simulink model "TEST_SensorSource_Lookup"  (R2020b)
settings: Solver=ode1  StartTime=tspan(1)  StopTime=tspan(2)  FixedStep=1/sensorFs.imuUpdateFs  RelTol=1e-3
values from neighbouring files (symbols this model uses):
  mag1 = double([Sensors.mag1.mag_x, Sensors.mag1.mag_y, Sensors.mag1.mag_z])    [navi_marg22.m]    (also in navi_marg24.m; navi_mvo17.m)
  mag2 = double([Sensors.mag2.mag_x, Sensors.mag2.mag_y, Sensors.mag2.mag_z])    [navi_marg22.m]    (also in navi_marg24.m; navi_mvo17.m)
  time = naviRes.time    [Plot_NaviMARG.m]    (also in UAVPlotLib.m = sensors.(sensorName).time; myplot_navfilter.m = sensors.Algo.time_algo; myplot_sensor_filter_compare.m = sensors.IMU.time_imu; postplot_marg_flightdata.m = sensors.Algo.time_algo)
undefined symbols (not defined in the file or in its folder): airspeed1, airspeed2, airspeed3, baro1, IMU1, IMU1_Control, IMU2, IMU3, laserDown1, laserDown2, radar1, radarLongDown1, radarLongForward1, sensorFs, ublox1, um482
(part 1 of 2)
settings Model: PauseTimes=266.88  Creator=sl  LastModifiedBy=sl
settings SolverCC: AutoInsertRateTranBlk=on
settings OptimizationCC: DefaultParameterBehavior=Inlined  EnhancedBackFolding=on  PassReuseOutputArgsAs=Individual arguments  ZeroExternalMemoryAtStartup=off  ZeroInternalMemoryAtStartup=off  MaxStackSize=64  OptimizeBlockOrder=speed  DifferentSizesBufferReuse=on  OptimizationCustomize=off  EfficientTunableParamExpr=on
settings DebuggingCC: MultiTaskCondExecSysMsg=none  ParameterPrecisionLossMsg=none  ParameterTunabilityLossMsg=error  UnconnectedInputMsg=none  UnconnectedOutputMsg=none  UnconnectedLineMsg=none  BusObjectLabelMismatch=error
settings HardwareCC: ProdBitPerPointer=32  ProdBitPerSizeT=32  ProdBitPerPtrDiffT=32  ProdLargestAtomicInteger=Long  ProdLargestAtomicFloat=Double  ProdWordSize=32  ProdHWDeviceType=ARM Compatible->ARM Cortex
settings ModelReferenceCC: EnableParallelModelReferenceBuilds=on  ParallelModelReferenceMATLABWorkerInit=Load Top Model
settings SFSimCC: MATLABDynamicMemAlloc=off
settings RTWCC: Description=Embedded Coder  SystemTargetFile=ert.tlc  TemplateMakefile=ert_default_tmf  GenerateReport=on  Toolchain=GNU Tools for ARM Embedded Processors  IncludeHyperlinkInReport=on  LaunchReport=on  GenerateTraceInfo=on  GenerateTraceReport=on  GenerateTraceReportSl=on  GenerateTraceReportSf=on  GenerateTraceReportEml=on
settings CodeAppCC: ForceParamTrailComments=on  IgnoreCustomStorageClasses=off  OperatorAnnotations=on  SimulinkDataObjDesc=on  SFDataObjDesc=on  InsertBlockDesc=on
settings ERTTargetCC: InlinedParameterPlacement=NonHierarchical  ERTCustomFileTemplate=example_file_process.tlc

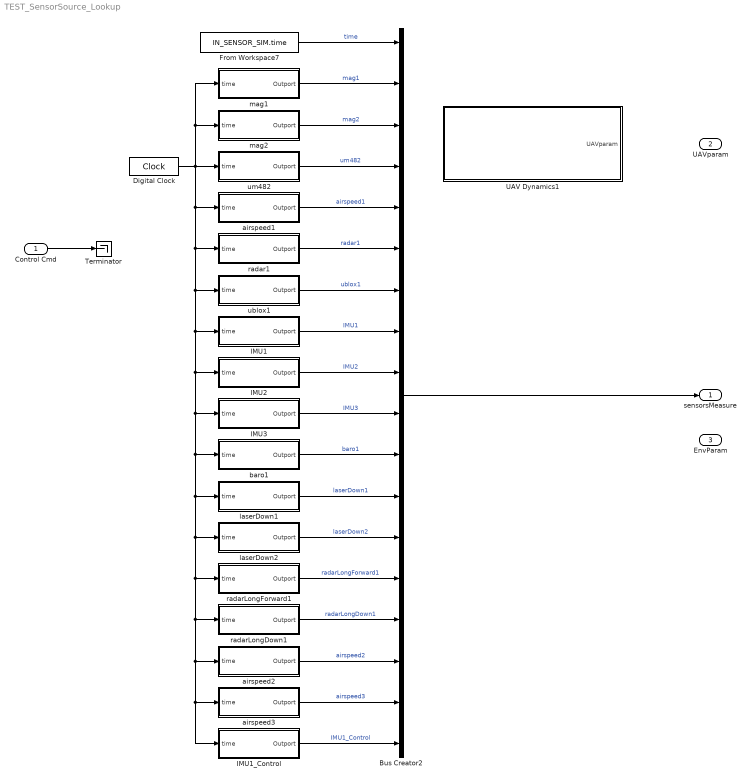
== system TEST_SensorSource_Lookup ==
  Control Cmd : Inport  OutDataTypeStr=Bus: BUS_CONTROL_ACTUATOR
  Bus Creator2 : BusCreator  Inputs=time,mag1,mag2,um482,airspeed1,radar1,ublox1,IMU1,IMU2,IMU3,baro1,laserDown1,laserDown2,radarLongForward1,radarLongDown1,airspeed2,airspeed3,IMU1_Control  OutDataTypeStr=Bus: BUS_SENSOR
  Digital Clock : DigitalClock  SampleTime=1/sensorFs.imuUpdateFs
  From Workspace7 : FromWorkspace  VariableName=IN_SENSOR_SIM.time  OutputAfterFinalValue=Holding final value
  IMU1 : Subsystem
  IMU1_Control : Subsystem
  IMU2 : Subsystem
  IMU3 : Subsystem
  Terminator : Terminator
  UAV Dynamics1 : Subsystem
  airspeed1 : Subsystem
  airspeed2 : Subsystem
  airspeed3 : Subsystem
  baro1 : Subsystem
  laserDown1 : Subsystem
  laserDown2 : Subsystem
  mag1 : Subsystem
  mag2 : Subsystem
  radar1 : Subsystem
  radarLongDown1 : Subsystem
  radarLongForward1 : Subsystem
  ublox1 : Subsystem
  um482 : Subsystem
  sensorsMeasure : Outport  OutDataTypeStr=Bus: BUS_SENSOR
  UAVparam : Outport  Port=2  OutDataTypeStr=Bus: BUS_UAVDYN_FlightParam
  EnvParam : Outport  Port=3  OutDataTypeStr=Bus: BUS_UAVDYN_Env  LockScale=on
  wires:
  um482/1(Outport) -> Bus Creator2/4  "um482"
  Control Cmd/1 -> Terminator/1
  radarLongForward1/1(Outport) -> Bus Creator2/14  "radarLongForward1"
  radar1/1(Outport) -> Bus Creator2/6  "radar1"
  mag2/1(Outport) -> Bus Creator2/3  "mag2"
  airspeed2/1(Outport) -> Bus Creator2/16  "airspeed2"
  IMU2/1(Outport) -> Bus Creator2/9  "IMU2"
  airspeed1/1(Outport) -> Bus Creator2/5  "airspeed1"
  radarLongDown1/1(Outport) -> Bus Creator2/15  "radarLongDown1"
  From Workspace7/1 -> Bus Creator2/1  "time"
  mag1/1(Outport) -> Bus Creator2/2  "mag1"
  IMU1/1(Outport) -> Bus Creator2/8  "IMU1"
  airspeed3/1(Outport) -> Bus Creator2/17  "airspeed3"
  Bus Creator2/1 -> sensorsMeasure/1
  IMU1_Control/1(Outport) -> Bus Creator2/18  "IMU1_Control"
  laserDown1/1(Outport) -> Bus Creator2/12  "laserDown1"
  baro1/1(Outport) -> Bus Creator2/11  "baro1"
  ublox1/1(Outport) -> Bus Creator2/7  "ublox1"
  laserDown2/1(Outport) -> Bus Creator2/13  "laserDown2"
  IMU3/1(Outport) -> Bus Creator2/10  "IMU3"
  Digital Clock/1 -> radarLongForward1/1(time), radarLongDown1/1(time), IMU1_Control/1(time), airspeed3/1(time), airspeed2/1(time), laserDown2/1(time), laserDown1/1(time), baro1/1(time), IMU3/1(time), IMU2/1(time), IMU1/1(time), ublox1/1(time), radar1/1(time), airspeed1/1(time), mag2/1(time), mag1/1(time), um482/1(time)

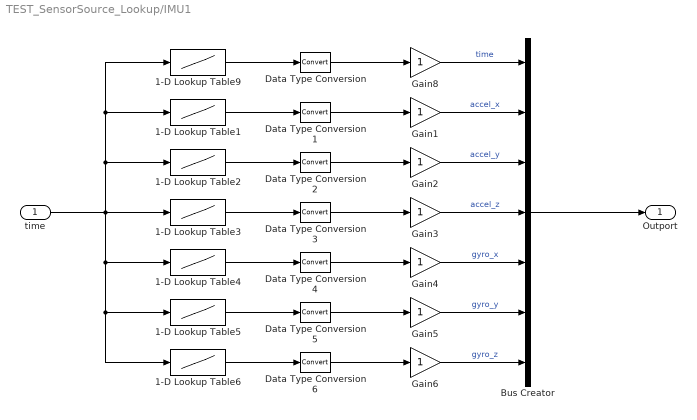
== system TEST_SensorSource_Lookup/IMU1 ==
  time : Inport
  1-D Lookup Table1 : Lookup_n-D  NumberOfTableDimensions=1  BreakpointsForDimension1=IN_SENSOR.IMU1.time(1:end-20)  Table=IN_SENSOR.IMU1.accel_x(1:end-20)  InterpMethod=Flat  ExtrapMethod=Clip  InternalRulePriority=Speed  RndMeth=Simplest  InputSameDT=on
  1-D Lookup Table2 : Lookup_n-D  NumberOfTableDimensions=1  BreakpointsForDimension1=IN_SENSOR.IMU1.time(1:end-20)  Table=IN_SENSOR.IMU1.accel_y(1:end-20)  InterpMethod=Flat  ExtrapMethod=Clip  InternalRulePriority=Speed  RndMeth=Simplest  InputSameDT=on
  1-D Lookup Table3 : Lookup_n-D  NumberOfTableDimensions=1  BreakpointsForDimension1=IN_SENSOR.IMU1.time(1:end-20)  Table=IN_SENSOR.IMU1.accel_z(1:end-20)  InterpMethod=Flat  ExtrapMethod=Clip  InternalRulePriority=Speed  RndMeth=Simplest  InputSameDT=on
  1-D Lookup Table4 : Lookup_n-D  NumberOfTableDimensions=1  BreakpointsForDimension1=IN_SENSOR.IMU1.time(1:end-20)  Table=IN_SENSOR.IMU1.gyro_x(1:end-20)  InterpMethod=Flat  ExtrapMethod=Clip  InternalRulePriority=Speed  RndMeth=Simplest  InputSameDT=on
  1-D Lookup Table5 : Lookup_n-D  NumberOfTableDimensions=1  BreakpointsForDimension1=IN_SENSOR.IMU1.time(1:end-20)  Table=IN_SENSOR.IMU1.gyro_y(1:end-20)  InterpMethod=Flat  ExtrapMethod=Clip  InternalRulePriority=Speed  RndMeth=Simplest  InputSameDT=on
  1-D Lookup Table6 : Lookup_n-D  NumberOfTableDimensions=1  BreakpointsForDimension1=IN_SENSOR.IMU1.time(1:end-20)  Table=IN_SENSOR.IMU1.gyro_z(1:end-20)  InterpMethod=Flat  ExtrapMethod=Clip  InternalRulePriority=Speed  RndMeth=Simplest  InputSameDT=on
  1-D Lookup Table9 : Lookup_n-D  NumberOfTableDimensions=1  BreakpointsForDimension1=IN_SENSOR.IMU1.time(1:end-20)  Table=IN_SENSOR.IMU1.time(1:end-20)  InterpMethod=Flat  ExtrapMethod=Clip  InternalRulePriority=Speed  RndMeth=Simplest  InputSameDT=on
  Bus Creator : BusCreator  Inputs=7
  Data Type Conversion{,1..6} (7 alike) : DataTypeConversion
  Gain{1..6,8} (7 alike) : Gain
  Outport : Outport
  wires:
  Gain2/1 -> Bus Creator/3  "accel_y"
  Gain6/1 -> Bus Creator/7  "gyro_z"
  Bus Creator/1 -> Outport/1
  Gain3/1 -> Bus Creator/4  "accel_z"
  Gain4/1 -> Bus Creator/5  "gyro_x"
  Gain1/1 -> Bus Creator/2  "accel_x"
  Gain8/1 -> Bus Creator/1  "time"
  Gain5/1 -> Bus Creator/6  "gyro_y"
  1-D Lookup Table9/1 -> Data Type Conversion/1
  Data Type Conversion/1 -> Gain8/1
  Data Type Conversion1/1 -> Gain1/1
  1-D Lookup Table1/1 -> Data Type Conversion1/1
  1-D Lookup Table2/1 -> Data Type Conversion2/1
  Data Type Conversion2/1 -> Gain2/1
  Data Type Conversion3/1 -> Gain3/1
  1-D Lookup Table3/1 -> Data Type Conversion3/1
  1-D Lookup Table4/1 -> Data Type Conversion4/1
  Data Type Conversion4/1 -> Gain4/1
  Data Type Conversion5/1 -> Gain5/1
  1-D Lookup Table5/1 -> Data Type Conversion5/1
  1-D Lookup Table6/1 -> Data Type Conversion6/1
  Data Type Conversion6/1 -> Gain6/1
  time/1 -> 1-D Lookup Table6/1, 1-D Lookup Table5/1, 1-D Lookup Table4/1, 1-D Lookup Table9/1, 1-D Lookup Table1/1, 1-D Lookup Table2/1, 1-D Lookup Table3/1

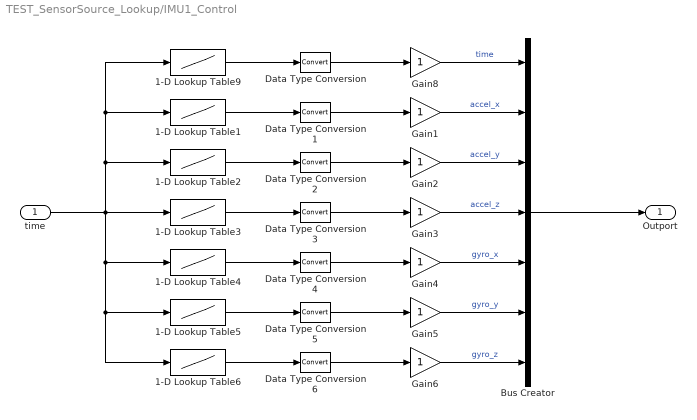
== system TEST_SensorSource_Lookup/IMU1_Control ==
  time : Inport
  1-D Lookup Table1 : Lookup_n-D  NumberOfTableDimensions=1  BreakpointsForDimension1=IN_SENSOR.IMU1_Control.time(1:end-20)  Table=IN_SENSOR.IMU1_Control.accel_x(1:end-20)  InterpMethod=Flat  ExtrapMethod=Clip  InternalRulePriority=Speed  RndMeth=Simplest  InputSameDT=on
  1-D Lookup Table2 : Lookup_n-D  NumberOfTableDimensions=1  BreakpointsForDimension1=IN_SENSOR.IMU1_Control.time(1:end-20)  Table=IN_SENSOR.IMU1_Control.accel_y(1:end-20)  InterpMethod=Flat  ExtrapMethod=Clip  InternalRulePriority=Speed  RndMeth=Simplest  InputSameDT=on
  1-D Lookup Table3 : Lookup_n-D  NumberOfTableDimensions=1  BreakpointsForDimension1=IN_SENSOR.IMU1_Control.time(1:end-20)  Table=IN_SENSOR.IMU1_Control.accel_z(1:end-20)  InterpMethod=Flat  ExtrapMethod=Clip  InternalRulePriority=Speed  RndMeth=Simplest  InputSameDT=on
  1-D Lookup Table4 : Lookup_n-D  NumberOfTableDimensions=1  BreakpointsForDimension1=IN_SENSOR.IMU1_Control.time(1:end-20)  Table=IN_SENSOR.IMU1_Control.gyro_x(1:end-20)  InterpMethod=Flat  ExtrapMethod=Clip  InternalRulePriority=Speed  RndMeth=Simplest  InputSameDT=on
  1-D Lookup Table5 : Lookup_n-D  NumberOfTableDimensions=1  BreakpointsForDimension1=IN_SENSOR.IMU1_Control.time(1:end-20)  Table=IN_SENSOR.IMU1_Control.gyro_y(1:end-20)  InterpMethod=Flat  ExtrapMethod=Clip  InternalRulePriority=Speed  RndMeth=Simplest  InputSameDT=on
  1-D Lookup Table6 : Lookup_n-D  NumberOfTableDimensions=1  BreakpointsForDimension1=IN_SENSOR.IMU1_Control.time(1:end-20)  Table=IN_SENSOR.IMU1_Control.gyro_z(1:end-20)  InterpMethod=Flat  ExtrapMethod=Clip  InternalRulePriority=Speed  RndMeth=Simplest  InputSameDT=on
  1-D Lookup Table9 : Lookup_n-D  NumberOfTableDimensions=1  BreakpointsForDimension1=IN_SENSOR.IMU1_Control.time(1:end-20)  Table=IN_SENSOR.IMU1_Control.time(1:end-20)  InterpMethod=Flat  ExtrapMethod=Clip  InternalRulePriority=Speed  RndMeth=Simplest  InputSameDT=on
  Bus Creator : BusCreator  Inputs=7
  Data Type Conversion{,1..6} (7 alike) : DataTypeConversion
  Gain{1..6,8} (7 alike) : Gain
  Outport : Outport
  wires:
  Gain2/1 -> Bus Creator/3  "accel_y"
  Gain6/1 -> Bus Creator/7  "gyro_z"
  Bus Creator/1 -> Outport/1
  Gain3/1 -> Bus Creator/4  "accel_z"
  Gain4/1 -> Bus Creator/5  "gyro_x"
  Gain1/1 -> Bus Creator/2  "accel_x"
  Gain8/1 -> Bus Creator/1  "time"
  Gain5/1 -> Bus Creator/6  "gyro_y"
  1-D Lookup Table9/1 -> Data Type Conversion/1
  Data Type Conversion/1 -> Gain8/1
  Data Type Conversion1/1 -> Gain1/1
  1-D Lookup Table1/1 -> Data Type Conversion1/1
  1-D Lookup Table2/1 -> Data Type Conversion2/1
  Data Type Conversion2/1 -> Gain2/1
  Data Type Conversion3/1 -> Gain3/1
  1-D Lookup Table3/1 -> Data Type Conversion3/1
  1-D Lookup Table4/1 -> Data Type Conversion4/1
  Data Type Conversion4/1 -> Gain4/1
  Data Type Conversion5/1 -> Gain5/1
  1-D Lookup Table5/1 -> Data Type Conversion5/1
  1-D Lookup Table6/1 -> Data Type Conversion6/1
  Data Type Conversion6/1 -> Gain6/1
  time/1 -> 1-D Lookup Table6/1, 1-D Lookup Table5/1, 1-D Lookup Table4/1, 1-D Lookup Table9/1, 1-D Lookup Table1/1, 1-D Lookup Table2/1, 1-D Lookup Table3/1

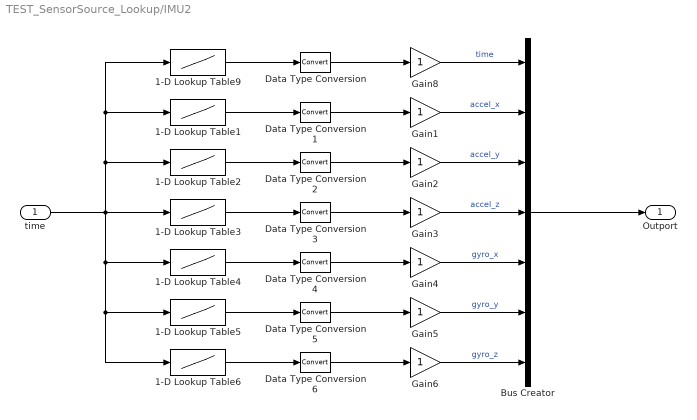
== system TEST_SensorSource_Lookup/IMU2 ==
  time : Inport
  1-D Lookup Table1 : Lookup_n-D  NumberOfTableDimensions=1  BreakpointsForDimension1=IN_SENSOR.IMU2.time(1:end-20)  Table=IN_SENSOR.IMU2.accel_x(1:end-20)  InterpMethod=Flat  ExtrapMethod=Clip  InternalRulePriority=Speed  RndMeth=Simplest  InputSameDT=on
  1-D Lookup Table2 : Lookup_n-D  NumberOfTableDimensions=1  BreakpointsForDimension1=IN_SENSOR.IMU2.time(1:end-20)  Table=IN_SENSOR.IMU2.accel_y(1:end-20)  InterpMethod=Flat  ExtrapMethod=Clip  InternalRulePriority=Speed  RndMeth=Simplest  InputSameDT=on
  1-D Lookup Table3 : Lookup_n-D  NumberOfTableDimensions=1  BreakpointsForDimension1=IN_SENSOR.IMU2.time(1:end-20)  Table=IN_SENSOR.IMU2.accel_z(1:end-20)  InterpMethod=Flat  ExtrapMethod=Clip  InternalRulePriority=Speed  RndMeth=Simplest  InputSameDT=on
  1-D Lookup Table4 : Lookup_n-D  NumberOfTableDimensions=1  BreakpointsForDimension1=IN_SENSOR.IMU2.time(1:end-20)  Table=IN_SENSOR.IMU2.gyro_x(1:end-20)  InterpMethod=Flat  ExtrapMethod=Clip  InternalRulePriority=Speed  RndMeth=Simplest  InputSameDT=on
  1-D Lookup Table5 : Lookup_n-D  NumberOfTableDimensions=1  BreakpointsForDimension1=IN_SENSOR.IMU2.time(1:end-20)  Table=IN_SENSOR.IMU2.gyro_y(1:end-20)  InterpMethod=Flat  ExtrapMethod=Clip  InternalRulePriority=Speed  RndMeth=Simplest  InputSameDT=on
  1-D Lookup Table6 : Lookup_n-D  NumberOfTableDimensions=1  BreakpointsForDimension1=IN_SENSOR.IMU2.time(1:end-20)  Table=IN_SENSOR.IMU2.gyro_z(1:end-20)  InterpMethod=Flat  ExtrapMethod=Clip  InternalRulePriority=Speed  RndMeth=Simplest  InputSameDT=on
  1-D Lookup Table9 : Lookup_n-D  NumberOfTableDimensions=1  BreakpointsForDimension1=IN_SENSOR.IMU2.time(1:end-20)  Table=IN_SENSOR.IMU2.time(1:end-20)  InterpMethod=Flat  ExtrapMethod=Clip  InternalRulePriority=Speed  RndMeth=Simplest  InputSameDT=on
  Bus Creator : BusCreator  Inputs=7
  Data Type Conversion{,1..6} (7 alike) : DataTypeConversion
  Gain{1..6,8} (7 alike) : Gain
  Outport : Outport
  wires:
  time/1 -> 1-D Lookup Table3/1, 1-D Lookup Table2/1, 1-D Lookup Table1/1, 1-D Lookup Table9/1, 1-D Lookup Table4/1, 1-D Lookup Table5/1, 1-D Lookup Table6/1
  Data Type Conversion6/1 -> Gain6/1
  1-D Lookup Table6/1 -> Data Type Conversion6/1
  1-D Lookup Table5/1 -> Data Type Conversion5/1
  Data Type Conversion5/1 -> Gain5/1
  Data Type Conversion4/1 -> Gain4/1
  1-D Lookup Table4/1 -> Data Type Conversion4/1
  1-D Lookup Table3/1 -> Data Type Conversion3/1
  Data Type Conversion3/1 -> Gain3/1
  Data Type Conversion2/1 -> Gain2/1
  1-D Lookup Table2/1 -> Data Type Conversion2/1
  1-D Lookup Table1/1 -> Data Type Conversion1/1
  Data Type Conversion1/1 -> Gain1/1
  Data Type Conversion/1 -> Gain8/1
  1-D Lookup Table9/1 -> Data Type Conversion/1
  Gain5/1 -> Bus Creator/6  "gyro_y"
  Gain8/1 -> Bus Creator/1  "time"
  Gain1/1 -> Bus Creator/2  "accel_x"
  Gain4/1 -> Bus Creator/5  "gyro_x"
  Gain3/1 -> Bus Creator/4  "accel_z"
  Bus Creator/1 -> Outport/1
  Gain6/1 -> Bus Creator/7  "gyro_z"
  Gain2/1 -> Bus Creator/3  "accel_y"

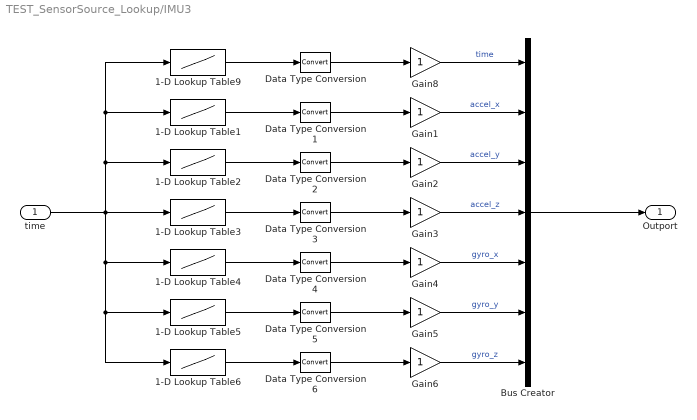
== system TEST_SensorSource_Lookup/IMU3 ==
  time : Inport
  1-D Lookup Table1 : Lookup_n-D  NumberOfTableDimensions=1  BreakpointsForDimension1=IN_SENSOR.IMU3.time(1:end-20)  Table=IN_SENSOR.IMU3.accel_x(1:end-20)  InterpMethod=Flat  ExtrapMethod=Clip  InternalRulePriority=Speed  RndMeth=Simplest  InputSameDT=on
  1-D Lookup Table2 : Lookup_n-D  NumberOfTableDimensions=1  BreakpointsForDimension1=IN_SENSOR.IMU3.time(1:end-20)  Table=IN_SENSOR.IMU3.accel_y(1:end-20)  InterpMethod=Flat  ExtrapMethod=Clip  InternalRulePriority=Speed  RndMeth=Simplest  InputSameDT=on
  1-D Lookup Table3 : Lookup_n-D  NumberOfTableDimensions=1  BreakpointsForDimension1=IN_SENSOR.IMU3.time(1:end-20)  Table=IN_SENSOR.IMU3.accel_z(1:end-20)  InterpMethod=Flat  ExtrapMethod=Clip  InternalRulePriority=Speed  RndMeth=Simplest  InputSameDT=on
  1-D Lookup Table4 : Lookup_n-D  NumberOfTableDimensions=1  BreakpointsForDimension1=IN_SENSOR.IMU3.time(1:end-20)  Table=IN_SENSOR.IMU3.gyro_x(1:end-20)  InterpMethod=Flat  ExtrapMethod=Clip  InternalRulePriority=Speed  RndMeth=Simplest  InputSameDT=on
  1-D Lookup Table5 : Lookup_n-D  NumberOfTableDimensions=1  BreakpointsForDimension1=IN_SENSOR.IMU3.time(1:end-20)  Table=IN_SENSOR.IMU3.gyro_y(1:end-20)  InterpMethod=Flat  ExtrapMethod=Clip  InternalRulePriority=Speed  RndMeth=Simplest  InputSameDT=on
  1-D Lookup Table6 : Lookup_n-D  NumberOfTableDimensions=1  BreakpointsForDimension1=IN_SENSOR.IMU3.time(1:end-20)  Table=IN_SENSOR.IMU3.gyro_z(1:end-20)  InterpMethod=Flat  ExtrapMethod=Clip  InternalRulePriority=Speed  RndMeth=Simplest  InputSameDT=on
  1-D Lookup Table9 : Lookup_n-D  NumberOfTableDimensions=1  BreakpointsForDimension1=IN_SENSOR.IMU3.time(1:end-20)  Table=IN_SENSOR.IMU3.time(1:end-20)  InterpMethod=Flat  ExtrapMethod=Clip  InternalRulePriority=Speed  RndMeth=Simplest  InputSameDT=on
  Bus Creator : BusCreator  Inputs=7
  Data Type Conversion{,1..6} (7 alike) : DataTypeConversion
  Gain{1..6,8} (7 alike) : Gain
  Outport : Outport
  wires:
  Gain2/1 -> Bus Creator/3  "accel_y"
  Gain6/1 -> Bus Creator/7  "gyro_z"
  Bus Creator/1 -> Outport/1
  Gain3/1 -> Bus Creator/4  "accel_z"
  Gain4/1 -> Bus Creator/5  "gyro_x"
  Gain1/1 -> Bus Creator/2  "accel_x"
  Gain8/1 -> Bus Creator/1  "time"
  Gain5/1 -> Bus Creator/6  "gyro_y"
  1-D Lookup Table9/1 -> Data Type Conversion/1
  Data Type Conversion/1 -> Gain8/1
  Data Type Conversion1/1 -> Gain1/1
  1-D Lookup Table1/1 -> Data Type Conversion1/1
  1-D Lookup Table2/1 -> Data Type Conversion2/1
  Data Type Conversion2/1 -> Gain2/1
  Data Type Conversion3/1 -> Gain3/1
  1-D Lookup Table3/1 -> Data Type Conversion3/1
  1-D Lookup Table4/1 -> Data Type Conversion4/1
  Data Type Conversion4/1 -> Gain4/1
  Data Type Conversion5/1 -> Gain5/1
  1-D Lookup Table5/1 -> Data Type Conversion5/1
  1-D Lookup Table6/1 -> Data Type Conversion6/1
  Data Type Conversion6/1 -> Gain6/1
  time/1 -> 1-D Lookup Table6/1, 1-D Lookup Table5/1, 1-D Lookup Table4/1, 1-D Lookup Table9/1, 1-D Lookup Table1/1, 1-D Lookup Table2/1, 1-D Lookup Table3/1

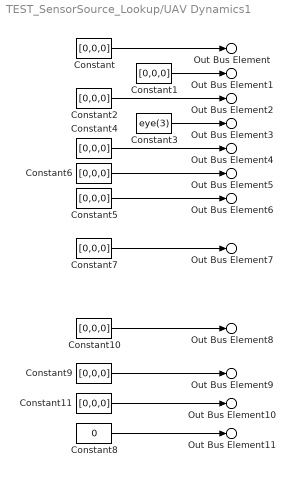
== system TEST_SensorSource_Lookup/UAV Dynamics1 ==
  Constant{,1..2,4..7,9..11} (10 alike) : Constant  Value=[0,0,0]
  Constant3 : Constant  Value=eye(3)
  Constant8 : Constant  Value=0
  Out Bus Element : Outport  PortName=UAVparam  Element=vel_NED
  Out Bus Element1 : Outport  PortName=UAVparam  Element=pos_NED
  Out Bus Element2 : Outport  PortName=UAVparam  Element=euler_yaw_pitch_roll
  Out Bus Element3 : Outport  PortName=UAVparam  Element=DCMbe
  Out Bus Element4 : Outport  PortName=UAVparam  Element=vel_Body
  Out Bus Element5 : Outport  PortName=UAVparam  Element=w_Body
  Out Bus Element6 : Outport  PortName=UAVparam  Element=dw_Body
  Out Bus Element7 : Outport  PortName=UAVparam  Element=LLA
  Out Bus Element8 : Outport  PortName=UAVparam  Element=specificForce_Body
  Out Bus Element9 : Outport  PortName=UAVparam  Element=mag_Body
  Out Bus Element10 : Outport  PortName=UAVparam  Element=mag_NED
  Out Bus Element11 : Outport  PortName=UAVparam  Element=magDec_deg
  wires:
  Constant/1 -> Out Bus Element/1
  Constant1/1 -> Out Bus Element1/1
  Constant2/1 -> Out Bus Element2/1
  Constant3/1 -> Out Bus Element3/1
  Constant4/1 -> Out Bus Element4/1
  Constant6/1 -> Out Bus Element5/1
  Constant5/1 -> Out Bus Element6/1
  Constant7/1 -> Out Bus Element7/1
  Constant10/1 -> Out Bus Element8/1
  Constant9/1 -> Out Bus Element9/1
  Constant11/1 -> Out Bus Element10/1
  Constant8/1 -> Out Bus Element11/1

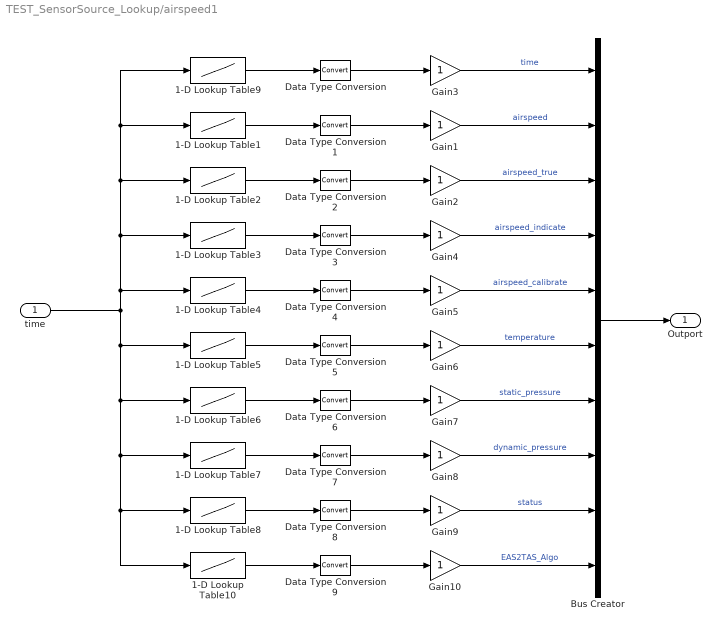
== system TEST_SensorSource_Lookup/airspeed1 ==
  time : Inport
  1-D Lookup Table1 : Lookup_n-D  NumberOfTableDimensions=1  BreakpointsForDimension1=IN_SENSOR.airspeed1.time(1:end-20)  Table=IN_SENSOR.airspeed1.airspeed(1:end-20)  InterpMethod=Flat  ExtrapMethod=Clip  InternalRulePriority=Speed  RndMeth=Simplest  InputSameDT=on
  1-D Lookup Table10 : Lookup_n-D  NumberOfTableDimensions=1  BreakpointsForDimension1=IN_SENSOR.airspeed1.time(1:end-20)  Table=IN_SENSOR.airspeed1.EAS2TAS_Algo(1:end-20)  InterpMethod=Flat  ExtrapMethod=Clip  InternalRulePriority=Speed  RndMeth=Simplest  InputSameDT=on
  1-D Lookup Table2 : Lookup_n-D  NumberOfTableDimensions=1  BreakpointsForDimension1=IN_SENSOR.airspeed1.time(1:end-20)  Table=IN_SENSOR.airspeed1.airspeed_true(1:end-20)  InterpMethod=Flat  ExtrapMethod=Clip  InternalRulePriority=Speed  RndMeth=Simplest  InputSameDT=on
  1-D Lookup Table3 : Lookup_n-D  NumberOfTableDimensions=1  BreakpointsForDimension1=IN_SENSOR.airspeed1.time(1:end-20)  Table=IN_SENSOR.airspeed1.airspeed_indicate(1:end-20)  InterpMethod=Flat  ExtrapMethod=Clip  InternalRulePriority=Speed  RndMeth=Simplest  InputSameDT=on
  1-D Lookup Table4 : Lookup_n-D  NumberOfTableDimensions=1  BreakpointsForDimension1=IN_SENSOR.airspeed1.time(1:end-20)  Table=IN_SENSOR.airspeed1.airspeed_calibrate(1:end-20)  InterpMethod=Flat  ExtrapMethod=Clip  InternalRulePriority=Speed  RndMeth=Simplest  InputSameDT=on
  1-D Lookup Table5 : Lookup_n-D  NumberOfTableDimensions=1  BreakpointsForDimension1=IN_SENSOR.airspeed1.time(1:end-20)  Table=IN_SENSOR.airspeed1.temperature(1:end-20)  InterpMethod=Flat  ExtrapMethod=Clip  InternalRulePriority=Speed  RndMeth=Simplest  InputSameDT=on
  1-D Lookup Table6 : Lookup_n-D  NumberOfTableDimensions=1  BreakpointsForDimension1=IN_SENSOR.airspeed1.time(1:end-20)  Table=IN_SENSOR.airspeed1.static_pressure(1:end-20)  InterpMethod=Flat  ExtrapMethod=Clip  InternalRulePriority=Speed  RndMeth=Simplest  InputSameDT=on
  1-D Lookup Table7 : Lookup_n-D  NumberOfTableDimensions=1  BreakpointsForDimension1=IN_SENSOR.airspeed1.time(1:end-20)  Table=IN_SENSOR.airspeed1.dynamic_pressure(1:end-20)  InterpMethod=Flat  ExtrapMethod=Clip  InternalRulePriority=Speed  RndMeth=Simplest  InputSameDT=on
  1-D Lookup Table8 : Lookup_n-D  NumberOfTableDimensions=1  BreakpointsForDimension1=IN_SENSOR.airspeed1.time(1:end-20)  Table=IN_SENSOR.airspeed1.status(1:end-20)  InterpMethod=Flat  ExtrapMethod=Clip  InternalRulePriority=Speed  RndMeth=Simplest  InputSameDT=on
  1-D Lookup Table9 : Lookup_n-D  NumberOfTableDimensions=1  BreakpointsForDimension1=IN_SENSOR.airspeed1.time(1:end-20)  Table=IN_SENSOR.airspeed1.time(1:end-20)  InterpMethod=Flat  ExtrapMethod=Clip  InternalRulePriority=Speed  RndMeth=Simplest  InputSameDT=on
  Bus Creator : BusCreator  Inputs=10
  Data Type Conversion{,1..9} (10 alike) : DataTypeConversion
  Gain{1..10} (10 alike) : Gain
  Outport : Outport
  wires:
  Bus Creator/1 -> Outport/1
  Gain1/1 -> Bus Creator/2  "airspeed"
  Gain3/1 -> Bus Creator/1  "time"
  Gain2/1 -> Bus Creator/3  "airspeed_true"
  Gain4/1 -> Bus Creator/4  "airspeed_indicate"
  Gain5/1 -> Bus Creator/5  "airspeed_calibrate"
  Gain6/1 -> Bus Creator/6  "temperature"
  Gain7/1 -> Bus Creator/7  "static_pressure"
  Gain8/1 -> Bus Creator/8  "dynamic_pressure"
  Gain9/1 -> Bus Creator/9  "status"
  Gain10/1 -> Bus Creator/10  "EAS2TAS_Algo"
  Data Type Conversion/1 -> Gain3/1
  1-D Lookup Table9/1 -> Data Type Conversion/1
  1-D Lookup Table1/1 -> Data Type Conversion1/1
  Data Type Conversion1/1 -> Gain1/1
  Data Type Conversion2/1 -> Gain2/1
  1-D Lookup Table2/1 -> Data Type Conversion2/1
  1-D Lookup Table3/1 -> Data Type Conversion3/1
  Data Type Conversion3/1 -> Gain4/1
  Data Type Conversion4/1 -> Gain5/1
  1-D Lookup Table4/1 -> Data Type Conversion4/1
  1-D Lookup Table5/1 -> Data Type Conversion5/1
  Data Type Conversion5/1 -> Gain6/1
  Data Type Conversion6/1 -> Gain7/1
  1-D Lookup Table6/1 -> Data Type Conversion6/1
  1-D Lookup Table7/1 -> Data Type Conversion7/1
  Data Type Conversion7/1 -> Gain8/1
  Data Type Conversion8/1 -> Gain9/1
  1-D Lookup Table8/1 -> Data Type Conversion8/1
  1-D Lookup Table10/1 -> Data Type Conversion9/1
  Data Type Conversion9/1 -> Gain10/1
  time/1 -> 1-D Lookup Table10/1, 1-D Lookup Table8/1, 1-D Lookup Table7/1, 1-D Lookup Table6/1, 1-D Lookup Table5/1, 1-D Lookup Table3/1, 1-D Lookup Table9/1, 1-D Lookup Table1/1, 1-D Lookup Table2/1, 1-D Lookup Table4/1

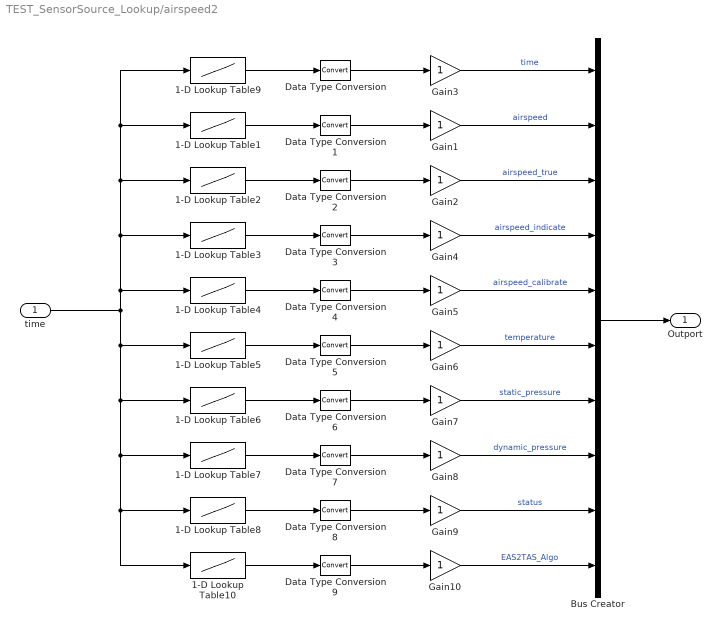
== system TEST_SensorSource_Lookup/airspeed2 ==
  time : Inport
  1-D Lookup Table1 : Lookup_n-D  NumberOfTableDimensions=1  BreakpointsForDimension1=IN_SENSOR.airspeed2.time(1:end-20)  Table=IN_SENSOR.airspeed2.airspeed(1:end-20)  InterpMethod=Flat  ExtrapMethod=Clip  InternalRulePriority=Speed  RndMeth=Simplest  InputSameDT=on
  1-D Lookup Table10 : Lookup_n-D  NumberOfTableDimensions=1  BreakpointsForDimension1=IN_SENSOR.airspeed2.time(1:end-20)  Table=IN_SENSOR.airspeed2.EAS2TAS_Algo(1:end-20)  InterpMethod=Flat  ExtrapMethod=Clip  InternalRulePriority=Speed  RndMeth=Simplest  InputSameDT=on
  1-D Lookup Table2 : Lookup_n-D  NumberOfTableDimensions=1  BreakpointsForDimension1=IN_SENSOR.airspeed2.time(1:end-20)  Table=IN_SENSOR.airspeed2.airspeed_true(1:end-20)  InterpMethod=Flat  ExtrapMethod=Clip  InternalRulePriority=Speed  RndMeth=Simplest  InputSameDT=on
  1-D Lookup Table3 : Lookup_n-D  NumberOfTableDimensions=1  BreakpointsForDimension1=IN_SENSOR.airspeed2.time(1:end-20)  Table=IN_SENSOR.airspeed2.airspeed_indicate(1:end-20)  InterpMethod=Flat  ExtrapMethod=Clip  InternalRulePriority=Speed  RndMeth=Simplest  InputSameDT=on
  1-D Lookup Table4 : Lookup_n-D  NumberOfTableDimensions=1  BreakpointsForDimension1=IN_SENSOR.airspeed2.time(1:end-20)  Table=IN_SENSOR.airspeed2.airspeed_calibrate(1:end-20)  InterpMethod=Flat  ExtrapMethod=Clip  InternalRulePriority=Speed  RndMeth=Simplest  InputSameDT=on
  1-D Lookup Table5 : Lookup_n-D  NumberOfTableDimensions=1  BreakpointsForDimension1=IN_SENSOR.airspeed2.time(1:end-20)  Table=IN_SENSOR.airspeed2.temperature(1:end-20)  InterpMethod=Flat  ExtrapMethod=Clip  InternalRulePriority=Speed  RndMeth=Simplest  InputSameDT=on
  1-D Lookup Table6 : Lookup_n-D  NumberOfTableDimensions=1  BreakpointsForDimension1=IN_SENSOR.airspeed2.time(1:end-20)  Table=IN_SENSOR.airspeed2.static_pressure(1:end-20)  InterpMethod=Flat  ExtrapMethod=Clip  InternalRulePriority=Speed  RndMeth=Simplest  InputSameDT=on
  1-D Lookup Table7 : Lookup_n-D  NumberOfTableDimensions=1  BreakpointsForDimension1=IN_SENSOR.airspeed2.time(1:end-20)  Table=IN_SENSOR.airspeed2.dynamic_pressure(1:end-20)  InterpMethod=Flat  ExtrapMethod=Clip  InternalRulePriority=Speed  RndMeth=Simplest  InputSameDT=on
  1-D Lookup Table8 : Lookup_n-D  NumberOfTableDimensions=1  BreakpointsForDimension1=IN_SENSOR.airspeed2.time(1:end-20)  Table=IN_SENSOR.airspeed2.status(1:end-20)  InterpMethod=Flat  ExtrapMethod=Clip  InternalRulePriority=Speed  RndMeth=Simplest  InputSameDT=on
  1-D Lookup Table9 : Lookup_n-D  NumberOfTableDimensions=1  BreakpointsForDimension1=IN_SENSOR.airspeed2.time(1:end-20)  Table=IN_SENSOR.airspeed2.time(1:end-20)  InterpMethod=Flat  ExtrapMethod=Clip  InternalRulePriority=Speed  RndMeth=Simplest  InputSameDT=on
  Bus Creator : BusCreator  Inputs=10
  Data Type Conversion{,1..9} (10 alike) : DataTypeConversion
  Gain{1..10} (10 alike) : Gain
  Outport : Outport
  wires:
  Bus Creator/1 -> Outport/1
  Gain1/1 -> Bus Creator/2  "airspeed"
  Gain3/1 -> Bus Creator/1  "time"
  Gain2/1 -> Bus Creator/3  "airspeed_true"
  Gain4/1 -> Bus Creator/4  "airspeed_indicate"
  Gain5/1 -> Bus Creator/5  "airspeed_calibrate"
  Gain6/1 -> Bus Creator/6  "temperature"
  Gain7/1 -> Bus Creator/7  "static_pressure"
  Gain8/1 -> Bus Creator/8  "dynamic_pressure"
  Gain9/1 -> Bus Creator/9  "status"
  Gain10/1 -> Bus Creator/10  "EAS2TAS_Algo"
  Data Type Conversion/1 -> Gain3/1
  1-D Lookup Table9/1 -> Data Type Conversion/1
  1-D Lookup Table1/1 -> Data Type Conversion1/1
  Data Type Conversion1/1 -> Gain1/1
  Data Type Conversion2/1 -> Gain2/1
  1-D Lookup Table2/1 -> Data Type Conversion2/1
  1-D Lookup Table3/1 -> Data Type Conversion3/1
  Data Type Conversion3/1 -> Gain4/1
  Data Type Conversion4/1 -> Gain5/1
  1-D Lookup Table4/1 -> Data Type Conversion4/1
  1-D Lookup Table5/1 -> Data Type Conversion5/1
  Data Type Conversion5/1 -> Gain6/1
  Data Type Conversion6/1 -> Gain7/1
  1-D Lookup Table6/1 -> Data Type Conversion6/1
  1-D Lookup Table7/1 -> Data Type Conversion7/1
  Data Type Conversion7/1 -> Gain8/1
  Data Type Conversion8/1 -> Gain9/1
  1-D Lookup Table8/1 -> Data Type Conversion8/1
  1-D Lookup Table10/1 -> Data Type Conversion9/1
  Data Type Conversion9/1 -> Gain10/1
  time/1 -> 1-D Lookup Table10/1, 1-D Lookup Table8/1, 1-D Lookup Table7/1, 1-D Lookup Table6/1, 1-D Lookup Table5/1, 1-D Lookup Table3/1, 1-D Lookup Table9/1, 1-D Lookup Table1/1, 1-D Lookup Table2/1, 1-D Lookup Table4/1

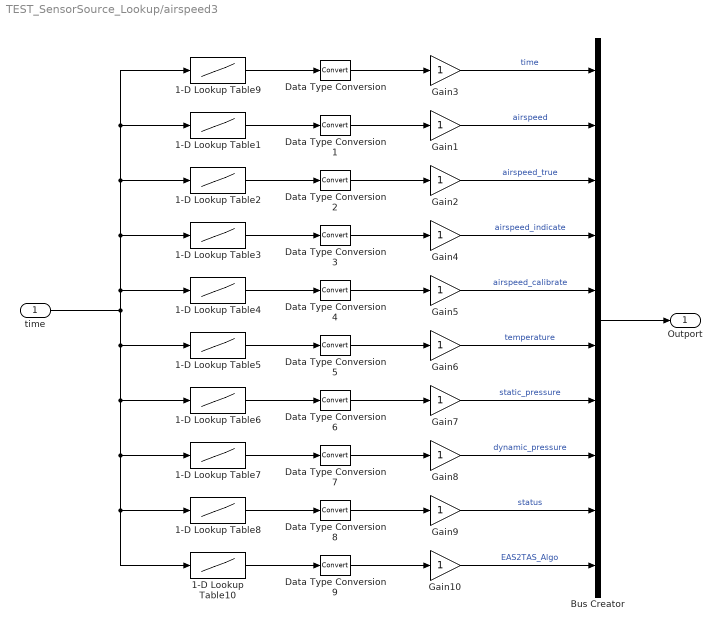
== system TEST_SensorSource_Lookup/airspeed3 ==
  time : Inport
  1-D Lookup Table1 : Lookup_n-D  NumberOfTableDimensions=1  BreakpointsForDimension1=IN_SENSOR.airspeed3.time(1:end-20)  Table=IN_SENSOR.airspeed3.airspeed(1:end-20)  InterpMethod=Flat  ExtrapMethod=Clip  InternalRulePriority=Speed  RndMeth=Simplest  InputSameDT=on
  1-D Lookup Table10 : Lookup_n-D  NumberOfTableDimensions=1  BreakpointsForDimension1=IN_SENSOR.airspeed3.time(1:end-20)  Table=IN_SENSOR.airspeed3.EAS2TAS_Algo(1:end-20)  InterpMethod=Flat  ExtrapMethod=Clip  InternalRulePriority=Speed  RndMeth=Simplest  InputSameDT=on
  1-D Lookup Table2 : Lookup_n-D  NumberOfTableDimensions=1  BreakpointsForDimension1=IN_SENSOR.airspeed3.time(1:end-20)  Table=IN_SENSOR.airspeed3.airspeed_true(1:end-20)  InterpMethod=Flat  ExtrapMethod=Clip  InternalRulePriority=Speed  RndMeth=Simplest  InputSameDT=on
  1-D Lookup Table3 : Lookup_n-D  NumberOfTableDimensions=1  BreakpointsForDimension1=IN_SENSOR.airspeed3.time(1:end-20)  Table=IN_SENSOR.airspeed3.airspeed_indicate(1:end-20)  InterpMethod=Flat  ExtrapMethod=Clip  InternalRulePriority=Speed  RndMeth=Simplest  InputSameDT=on
  1-D Lookup Table4 : Lookup_n-D  NumberOfTableDimensions=1  BreakpointsForDimension1=IN_SENSOR.airspeed3.time(1:end-20)  Table=IN_SENSOR.airspeed3.airspeed_calibrate(1:end-20)  InterpMethod=Flat  ExtrapMethod=Clip  InternalRulePriority=Speed  RndMeth=Simplest  InputSameDT=on
  1-D Lookup Table5 : Lookup_n-D  NumberOfTableDimensions=1  BreakpointsForDimension1=IN_SENSOR.airspeed3.time(1:end-20)  Table=IN_SENSOR.airspeed3.temperature(1:end-20)  InterpMethod=Flat  ExtrapMethod=Clip  InternalRulePriority=Speed  RndMeth=Simplest  InputSameDT=on
  1-D Lookup Table6 : Lookup_n-D  NumberOfTableDimensions=1  BreakpointsForDimension1=IN_SENSOR.airspeed3.time(1:end-20)  Table=IN_SENSOR.airspeed3.static_pressure(1:end-20)  InterpMethod=Flat  ExtrapMethod=Clip  InternalRulePriority=Speed  RndMeth=Simplest  InputSameDT=on
  1-D Lookup Table7 : Lookup_n-D  NumberOfTableDimensions=1  BreakpointsForDimension1=IN_SENSOR.airspeed3.time(1:end-20)  Table=IN_SENSOR.airspeed3.dynamic_pressure(1:end-20)  InterpMethod=Flat  ExtrapMethod=Clip  InternalRulePriority=Speed  RndMeth=Simplest  InputSameDT=on
  1-D Lookup Table8 : Lookup_n-D  NumberOfTableDimensions=1  BreakpointsForDimension1=IN_SENSOR.airspeed3.time(1:end-20)  Table=IN_SENSOR.airspeed3.status(1:end-20)  InterpMethod=Flat  ExtrapMethod=Clip  InternalRulePriority=Speed  RndMeth=Simplest  InputSameDT=on
  1-D Lookup Table9 : Lookup_n-D  NumberOfTableDimensions=1  BreakpointsForDimension1=IN_SENSOR.airspeed3.time(1:end-20)  Table=IN_SENSOR.airspeed3.time(1:end-20)  InterpMethod=Flat  ExtrapMethod=Clip  InternalRulePriority=Speed  RndMeth=Simplest  InputSameDT=on
  Bus Creator : BusCreator  Inputs=10
  Data Type Conversion{,1..9} (10 alike) : DataTypeConversion
  Gain{1..10} (10 alike) : Gain
  Outport : Outport
  wires:
  time/1 -> 1-D Lookup Table4/1, 1-D Lookup Table2/1, 1-D Lookup Table1/1, 1-D Lookup Table9/1, 1-D Lookup Table3/1, 1-D Lookup Table5/1, 1-D Lookup Table6/1, 1-D Lookup Table7/1, 1-D Lookup Table8/1, 1-D Lookup Table10/1
  Data Type Conversion9/1 -> Gain10/1
  1-D Lookup Table10/1 -> Data Type Conversion9/1
  1-D Lookup Table8/1 -> Data Type Conversion8/1
  Data Type Conversion8/1 -> Gain9/1
  Data Type Conversion7/1 -> Gain8/1
  1-D Lookup Table7/1 -> Data Type Conversion7/1
  1-D Lookup Table6/1 -> Data Type Conversion6/1
  Data Type Conversion6/1 -> Gain7/1
  Data Type Conversion5/1 -> Gain6/1
  1-D Lookup Table5/1 -> Data Type Conversion5/1
  1-D Lookup Table4/1 -> Data Type Conversion4/1
  Data Type Conversion4/1 -> Gain5/1
  Data Type Conversion3/1 -> Gain4/1
  1-D Lookup Table3/1 -> Data Type Conversion3/1
  1-D Lookup Table2/1 -> Data Type Conversion2/1
  Data Type Conversion2/1 -> Gain2/1
  Data Type Conversion1/1 -> Gain1/1
  1-D Lookup Table1/1 -> Data Type Conversion1/1
  1-D Lookup Table9/1 -> Data Type Conversion/1
  Data Type Conversion/1 -> Gain3/1
  Gain10/1 -> Bus Creator/10  "EAS2TAS_Algo"
  Gain9/1 -> Bus Creator/9  "status"
  Gain8/1 -> Bus Creator/8  "dynamic_pressure"
  Gain7/1 -> Bus Creator/7  "static_pressure"
  Gain6/1 -> Bus Creator/6  "temperature"
  Gain5/1 -> Bus Creator/5  "airspeed_calibrate"
  Gain4/1 -> Bus Creator/4  "airspeed_indicate"
  Gain2/1 -> Bus Creator/3  "airspeed_true"
  Gain3/1 -> Bus Creator/1  "time"
  Gain1/1 -> Bus Creator/2  "airspeed"
  Bus Creator/1 -> Outport/1

== system TEST_SensorSource_Lookup/baro1 ==
  time : Inport
  1-D Lookup Table1 : Lookup_n-D  NumberOfTableDimensions=1  BreakpointsForDimension1=IN_SENSOR.baro1.time(1:end-20)  Table=IN_SENSOR.baro1.alt_baro(1:end-20)  InterpMethod=Flat  ExtrapMethod=Clip  InternalRulePriority=Speed  RndMeth=Simplest  InputSameDT=on
  1-D Lookup Table9 : Lookup_n-D  NumberOfTableDimensions=1  BreakpointsForDimension1=IN_SENSOR.baro1.time(1:end-20)  Table=IN_SENSOR.baro1.time(1:end-20)  InterpMethod=Flat  ExtrapMethod=Clip  InternalRulePriority=Speed  RndMeth=Simplest  InputSameDT=on
  Bus Creator : BusCreator  Inputs=2
  Data Type Conversion : DataTypeConversion
  Data Type Conversion1 : DataTypeConversion
  Gain1 : Gain
  Gain8 : Gain
  Outport : Outport
  wires:
  Gain8/1 -> Bus Creator/1  "time"
  Gain1/1 -> Bus Creator/2  "alt_baro"
  Bus Creator/1 -> Outport/1
  Data Type Conversion/1 -> Gain8/1
  1-D Lookup Table9/1 -> Data Type Conversion/1
  1-D Lookup Table1/1 -> Data Type Conversion1/1
  Data Type Conversion1/1 -> Gain1/1
  time/1 -> 1-D Lookup Table1/1, 1-D Lookup Table9/1

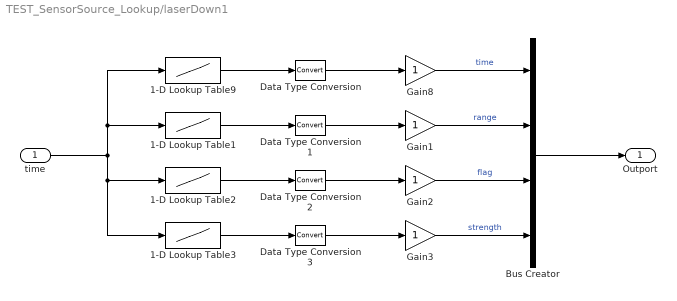
== system TEST_SensorSource_Lookup/laserDown1 ==
  time : Inport
  1-D Lookup Table1 : Lookup_n-D  NumberOfTableDimensions=1  BreakpointsForDimension1=IN_SENSOR.laserDown1.time(1:end-20)  Table=IN_SENSOR.laserDown1.range(1:end-20)  InterpMethod=Flat  ExtrapMethod=Clip  InternalRulePriority=Speed  RndMeth=Simplest  InputSameDT=on
  1-D Lookup Table2 : Lookup_n-D  NumberOfTableDimensions=1  BreakpointsForDimension1=IN_SENSOR.laserDown1.time(1:end-20)  Table=IN_SENSOR.laserDown1.flag(1:end-20)  InterpMethod=Flat  ExtrapMethod=Clip  InternalRulePriority=Speed  RndMeth=Simplest  InputSameDT=on
  1-D Lookup Table3 : Lookup_n-D  NumberOfTableDimensions=1  BreakpointsForDimension1=IN_SENSOR.laserDown1.time(1:end-20)  Table=IN_SENSOR.laserDown1.strength(1:end-20)  InterpMethod=Flat  ExtrapMethod=Clip  InternalRulePriority=Speed  RndMeth=Simplest  InputSameDT=on
  1-D Lookup Table9 : Lookup_n-D  NumberOfTableDimensions=1  BreakpointsForDimension1=IN_SENSOR.laserDown1.time(1:end-20)  Table=IN_SENSOR.laserDown1.time(1:end-20)  InterpMethod=Flat  ExtrapMethod=Clip  InternalRulePriority=Speed  RndMeth=Simplest  InputSameDT=on
  Bus Creator : BusCreator  Inputs=4
  Data Type Conversion{,1..3} (4 alike) : DataTypeConversion
  Gain{1..3,8} (4 alike) : Gain
  Outport : Outport
  wires:
  time/1 -> 1-D Lookup Table1/1, 1-D Lookup Table9/1, 1-D Lookup Table2/1, 1-D Lookup Table3/1
  1-D Lookup Table3/1 -> Data Type Conversion3/1
  Data Type Conversion3/1 -> Gain3/1
  Data Type Conversion2/1 -> Gain2/1
  1-D Lookup Table2/1 -> Data Type Conversion2/1
  1-D Lookup Table1/1 -> Data Type Conversion1/1
  Data Type Conversion1/1 -> Gain1/1
  Data Type Conversion/1 -> Gain8/1
  1-D Lookup Table9/1 -> Data Type Conversion/1
  Gain3/1 -> Bus Creator/4  "strength"
  Gain2/1 -> Bus Creator/3  "flag"
  Gain8/1 -> Bus Creator/1  "time"
  Gain1/1 -> Bus Creator/2  "range"
  Bus Creator/1 -> Outport/1

== system TEST_SensorSource_Lookup/laserDown2 ==
  time : Inport
  1-D Lookup Table1 : Lookup_n-D  NumberOfTableDimensions=1  BreakpointsForDimension1=IN_SENSOR.laserDown2.time(1:end-20)  Table=IN_SENSOR.laserDown2.range(1:end-20)  InterpMethod=Flat  ExtrapMethod=Clip  InternalRulePriority=Speed  RndMeth=Simplest  InputSameDT=on
  1-D Lookup Table2 : Lookup_n-D  NumberOfTableDimensions=1  BreakpointsForDimension1=IN_SENSOR.laserDown2.time(1:end-20)  Table=IN_SENSOR.laserDown2.flag(1:end-20)  InterpMethod=Flat  ExtrapMethod=Clip  InternalRulePriority=Speed  RndMeth=Simplest  InputSameDT=on
  1-D Lookup Table3 : Lookup_n-D  NumberOfTableDimensions=1  BreakpointsForDimension1=IN_SENSOR.laserDown2.time(1:end-20)  Table=IN_SENSOR.laserDown2.strength(1:end-20)  InterpMethod=Flat  ExtrapMethod=Clip  InternalRulePriority=Speed  RndMeth=Simplest  InputSameDT=on
  1-D Lookup Table9 : Lookup_n-D  NumberOfTableDimensions=1  BreakpointsForDimension1=IN_SENSOR.laserDown2.time(1:end-20)  Table=IN_SENSOR.laserDown2.time(1:end-20)  InterpMethod=Flat  ExtrapMethod=Clip  InternalRulePriority=Speed  RndMeth=Simplest  InputSameDT=on
  Bus Creator : BusCreator  Inputs=4
  Data Type Conversion{,1..3} (4 alike) : DataTypeConversion
  Gain{1..3,8} (4 alike) : Gain
  Outport : Outport
  wires:
  time/1 -> 1-D Lookup Table1/1, 1-D Lookup Table9/1, 1-D Lookup Table2/1, 1-D Lookup Table3/1
  1-D Lookup Table3/1 -> Data Type Conversion3/1
  Data Type Conversion3/1 -> Gain3/1
  Data Type Conversion2/1 -> Gain2/1
  1-D Lookup Table2/1 -> Data Type Conversion2/1
  1-D Lookup Table1/1 -> Data Type Conversion1/1
  Data Type Conversion1/1 -> Gain1/1
  Data Type Conversion/1 -> Gain8/1
  1-D Lookup Table9/1 -> Data Type Conversion/1
  Gain3/1 -> Bus Creator/4  "strength"
  Gain2/1 -> Bus Creator/3  "flag"
  Gain8/1 -> Bus Creator/1  "time"
  Gain1/1 -> Bus Creator/2  "range"
  Bus Creator/1 -> Outport/1

== system TEST_SensorSource_Lookup/mag1 ==
  time : Inport
  1-D Lookup Table1 : Lookup_n-D  NumberOfTableDimensions=1  BreakpointsForDimension1=IN_SENSOR.mag1.time(1:end-20)  Table=IN_SENSOR.mag1.mag_x(1:end-20)  InterpMethod=Flat  ExtrapMethod=Clip  InternalRulePriority=Speed  RndMeth=Simplest  InputSameDT=on
  1-D Lookup Table2 : Lookup_n-D  NumberOfTableDimensions=1  BreakpointsForDimension1=IN_SENSOR.mag1.time(1:end-20)  Table=IN_SENSOR.mag1.mag_y(1:end-20)  InterpMethod=Flat  ExtrapMethod=Clip  InternalRulePriority=Speed  RndMeth=Simplest  InputSameDT=on
  1-D Lookup Table3 : Lookup_n-D  NumberOfTableDimensions=1  BreakpointsForDimension1=IN_SENSOR.mag1.time(1:end-20)  Table=IN_SENSOR.mag1.mag_z(1:end-20)  InterpMethod=Flat  ExtrapMethod=Clip  InternalRulePriority=Speed  RndMeth=Simplest  InputSameDT=on
  1-D Lookup Table9 : Lookup_n-D  NumberOfTableDimensions=1  BreakpointsForDimension1=IN_SENSOR.mag1.time(1:end-20)  Table=IN_SENSOR.mag1.time(1:end-20)  InterpMethod=Flat  ExtrapMethod=Clip  InternalRulePriority=Speed  RndMeth=Simplest  InputSameDT=on
  Bus Creator : BusCreator  Inputs=4
  Data Type Conversion{,1..3} (4 alike) : DataTypeConversion
  Gain{1..4} (4 alike) : Gain
  Outport : Outport
  wires:
  Gain3/1 -> Bus Creator/1  "time"
  Gain1/1 -> Bus Creator/2  "mag_x"
  Gain4/1 -> Bus Creator/4  "mag_z"
  Bus Creator/1 -> Outport/1
  Gain2/1 -> Bus Creator/3  "mag_y"
  Data Type Conversion/1 -> Gain3/1
  1-D Lookup Table9/1 -> Data Type Conversion/1
  1-D Lookup Table1/1 -> Data Type Conversion1/1
  Data Type Conversion1/1 -> Gain1/1
  Data Type Conversion2/1 -> Gain2/1
  1-D Lookup Table2/1 -> Data Type Conversion2/1
  1-D Lookup Table3/1 -> Data Type Conversion3/1
  Data Type Conversion3/1 -> Gain4/1
  time/1 -> 1-D Lookup Table3/1, 1-D Lookup Table2/1, 1-D Lookup Table1/1, 1-D Lookup Table9/1

== system TEST_SensorSource_Lookup/mag2 ==
  time : Inport
  1-D Lookup Table1 : Lookup_n-D  NumberOfTableDimensions=1  BreakpointsForDimension1=IN_SENSOR.mag2.time(1:end-20)  Table=IN_SENSOR.mag2.mag_x(1:end-20)  InterpMethod=Flat  ExtrapMethod=Clip  InternalRulePriority=Speed  RndMeth=Simplest  InputSameDT=on
  1-D Lookup Table2 : Lookup_n-D  NumberOfTableDimensions=1  BreakpointsForDimension1=IN_SENSOR.mag2.time(1:end-20)  Table=IN_SENSOR.mag2.mag_y(1:end-20)  InterpMethod=Flat  ExtrapMethod=Clip  InternalRulePriority=Speed  RndMeth=Simplest  InputSameDT=on
  1-D Lookup Table3 : Lookup_n-D  NumberOfTableDimensions=1  BreakpointsForDimension1=IN_SENSOR.mag2.time(1:end-20)  Table=IN_SENSOR.mag2.mag_z(1:end-20)  InterpMethod=Flat  ExtrapMethod=Clip  InternalRulePriority=Speed  RndMeth=Simplest  InputSameDT=on
  1-D Lookup Table9 : Lookup_n-D  NumberOfTableDimensions=1  BreakpointsForDimension1=IN_SENSOR.mag2.time(1:end-20)  Table=IN_SENSOR.mag2.time(1:end-20)  InterpMethod=Flat  ExtrapMethod=Clip  InternalRulePriority=Speed  RndMeth=Simplest  InputSameDT=on
  Bus Creator : BusCreator  Inputs=4
  Data Type Conversion{,1..3} (4 alike) : DataTypeConversion
  Gain{1..4} (4 alike) : Gain
  Outport : Outport
  wires:
  time/1 -> 1-D Lookup Table9/1, 1-D Lookup Table1/1, 1-D Lookup Table2/1, 1-D Lookup Table3/1
  Data Type Conversion3/1 -> Gain4/1
  1-D Lookup Table3/1 -> Data Type Conversion3/1
  1-D Lookup Table2/1 -> Data Type Conversion2/1
  Data Type Conversion2/1 -> Gain2/1
  Data Type Conversion1/1 -> Gain1/1
  1-D Lookup Table1/1 -> Data Type Conversion1/1
  1-D Lookup Table9/1 -> Data Type Conversion/1
  Data Type Conversion/1 -> Gain3/1
  Gain2/1 -> Bus Creator/3  "mag_y"
  Bus Creator/1 -> Outport/1
  Gain4/1 -> Bus Creator/4  "mag_z"
  Gain1/1 -> Bus Creator/2  "mag_x"
  Gain3/1 -> Bus Creator/1  "time"

== system TEST_SensorSource_Lookup/radar1 ==
  time : Inport
  1-D Lookup Table1 : Lookup_n-D  NumberOfTableDimensions=1  BreakpointsForDimension1=IN_SENSOR.radar1.time(1:end-20)  Table=IN_SENSOR.radar1.SNR(1:end-20)  InterpMethod=Flat  ExtrapMethod=Clip  InternalRulePriority=Speed  RndMeth=Simplest  InputSameDT=on
  1-D Lookup Table2 : Lookup_n-D  NumberOfTableDimensions=1  BreakpointsForDimension1=IN_SENSOR.radar1.time(1:end-20)  Table=IN_SENSOR.radar1.Flag(1:end-20)  InterpMethod=Flat  ExtrapMethod=Clip  InternalRulePriority=Speed  RndMeth=Simplest  InputSameDT=on
  1-D Lookup Table3 : Lookup_n-D  NumberOfTableDimensions=1  BreakpointsForDimension1=IN_SENSOR.radar1.time(1:end-20)  Table=IN_SENSOR.radar1.Range(1:end-20)  InterpMethod=Flat  ExtrapMethod=Clip  InternalRulePriority=Speed  RndMeth=Simplest  InputSameDT=on
  1-D Lookup Table9 : Lookup_n-D  NumberOfTableDimensions=1  BreakpointsForDimension1=IN_SENSOR.radar1.time(1:end-20)  Table=IN_SENSOR.radar1.time(1:end-20)  InterpMethod=Flat  ExtrapMethod=Clip  InternalRulePriority=Speed  RndMeth=Simplest  InputSameDT=on
  Bus Creator : BusCreator  Inputs=4
  Data Type Conversion{,1..3} (4 alike) : DataTypeConversion
  Gain{1..4} (4 alike) : Gain
  Outport : Outport
  wires:
  Gain3/1 -> Bus Creator/1  "time"
  Gain1/1 -> Bus Creator/2  "SNR"
  Gain4/1 -> Bus Creator/4  "Range"
  Bus Creator/1 -> Outport/1
  Gain2/1 -> Bus Creator/3  "Flag"
  1-D Lookup Table9/1 -> Data Type Conversion/1
  Data Type Conversion/1 -> Gain3/1
  Data Type Conversion1/1 -> Gain1/1
  1-D Lookup Table1/1 -> Data Type Conversion1/1
  1-D Lookup Table2/1 -> Data Type Conversion2/1
  Data Type Conversion2/1 -> Gain2/1
  Data Type Conversion3/1 -> Gain4/1
  1-D Lookup Table3/1 -> Data Type Conversion3/1
  time/1 -> 1-D Lookup Table3/1, 1-D Lookup Table2/1, 1-D Lookup Table1/1, 1-D Lookup Table9/1

== system TEST_SensorSource_Lookup/radarLongDown1 ==
  time : Inport
  1-D Lookup Table1 : Lookup_n-D  NumberOfTableDimensions=1  BreakpointsForDimension1=IN_SENSOR.radarLongDown1.time(1:end-20)  Table=IN_SENSOR.radarLongDown1.range(1:end-20)  InterpMethod=Flat  ExtrapMethod=Clip  InternalRulePriority=Speed  RndMeth=Simplest  InputSameDT=on
  1-D Lookup Table2 : Lookup_n-D  NumberOfTableDimensions=1  BreakpointsForDimension1=IN_SENSOR.radarLongDown1.time(1:end-20)  Table=IN_SENSOR.radarLongDown1.flag(1:end-20)  InterpMethod=Flat  ExtrapMethod=Clip  InternalRulePriority=Speed  RndMeth=Simplest  InputSameDT=on
  1-D Lookup Table3 : Lookup_n-D  NumberOfTableDimensions=1  BreakpointsForDimension1=IN_SENSOR.radarLongDown1.time(1:end-20)  Table=IN_SENSOR.radarLongDown1.strength(1:end-20)  InterpMethod=Flat  ExtrapMethod=Clip  InternalRulePriority=Speed  RndMeth=Simplest  InputSameDT=on
  1-D Lookup Table9 : Lookup_n-D  NumberOfTableDimensions=1  BreakpointsForDimension1=IN_SENSOR.radarLongDown1.time(1:end-20)  Table=IN_SENSOR.radarLongDown1.time(1:end-20)  InterpMethod=Flat  ExtrapMethod=Clip  InternalRulePriority=Speed  RndMeth=Simplest  InputSameDT=on
  Bus Creator : BusCreator  Inputs=4
  Data Type Conversion{,1..3} (4 alike) : DataTypeConversion
  Gain{1..3,8} (4 alike) : Gain
  Outport : Outport
  wires:
  Bus Creator/1 -> Outport/1
  Gain1/1 -> Bus Creator/2  "range"
  Gain8/1 -> Bus Creator/1  "time"
  Gain2/1 -> Bus Creator/3  "flag"
  Gain3/1 -> Bus Creator/4  "strength"
  1-D Lookup Table9/1 -> Data Type Conversion/1
  Data Type Conversion/1 -> Gain8/1
  Data Type Conversion1/1 -> Gain1/1
  1-D Lookup Table1/1 -> Data Type Conversion1/1
  1-D Lookup Table2/1 -> Data Type Conversion2/1
  Data Type Conversion2/1 -> Gain2/1
  Data Type Conversion3/1 -> Gain3/1
  1-D Lookup Table3/1 -> Data Type Conversion3/1
  time/1 -> 1-D Lookup Table3/1, 1-D Lookup Table2/1, 1-D Lookup Table9/1, 1-D Lookup Table1/1

== system TEST_SensorSource_Lookup/radarLongForward1 ==
  time : Inport
  1-D Lookup Table1 : Lookup_n-D  NumberOfTableDimensions=1  BreakpointsForDimension1=IN_SENSOR.radarLongForward1.time(1:end-20)  Table=IN_SENSOR.radarLongForward1.range(1:end-20)  InterpMethod=Flat  ExtrapMethod=Clip  InternalRulePriority=Speed  RndMeth=Simplest  InputSameDT=on
  1-D Lookup Table2 : Lookup_n-D  NumberOfTableDimensions=1  BreakpointsForDimension1=IN_SENSOR.radarLongForward1.time(1:end-20)  Table=IN_SENSOR.radarLongForward1.flag(1:end-20)  InterpMethod=Flat  ExtrapMethod=Clip  InternalRulePriority=Speed  RndMeth=Simplest  InputSameDT=on
  1-D Lookup Table3 : Lookup_n-D  NumberOfTableDimensions=1  BreakpointsForDimension1=IN_SENSOR.radarLongForward1.time(1:end-20)  Table=IN_SENSOR.radarLongForward1.strength(1:end-20)  InterpMethod=Flat  ExtrapMethod=Clip  InternalRulePriority=Speed  RndMeth=Simplest  InputSameDT=on
  1-D Lookup Table9 : Lookup_n-D  NumberOfTableDimensions=1  BreakpointsForDimension1=IN_SENSOR.radarLongForward1.time(1:end-20)  Table=IN_SENSOR.radarLongForward1.time(1:end-20)  InterpMethod=Flat  ExtrapMethod=Clip  InternalRulePriority=Speed  RndMeth=Simplest  InputSameDT=on
  Bus Creator : BusCreator  Inputs=4
  Data Type Conversion{,1..3} (4 alike) : DataTypeConversion
  Gain{1..3,8} (4 alike) : Gain
  Outport : Outport
  wires:
  time/1 -> 1-D Lookup Table1/1, 1-D Lookup Table9/1, 1-D Lookup Table2/1, 1-D Lookup Table3/1
  1-D Lookup Table3/1 -> Data Type Conversion3/1
  Data Type Conversion3/1 -> Gain3/1
  Data Type Conversion2/1 -> Gain2/1
  1-D Lookup Table2/1 -> Data Type Conversion2/1
  1-D Lookup Table1/1 -> Data Type Conversion1/1
  Data Type Conversion1/1 -> Gain1/1
  Data Type Conversion/1 -> Gain8/1
  1-D Lookup Table9/1 -> Data Type Conversion/1
  Gain3/1 -> Bus Creator/4  "strength"
  Gain2/1 -> Bus Creator/3  "flag"
  Gain8/1 -> Bus Creator/1  "time"
  Gain1/1 -> Bus Creator/2  "range"
  Bus Creator/1 -> Outport/1
